simulink model "soc_WLAN_fpga"  (R2024b)
settings: Solver=FixedStepDiscrete  StartTime=0.0  StopTime=stopTime  RelTol=1e-3
PreLoadFcn:
  | addpath(fullfile(matlabroot,'toolbox','whdl','whdlexamples','whdlexamples'));
InitFcn:
  | addpath(fullfile(matlabroot,'toolbox','whdl','whdlexamples','whdlexamples'));
model workspace (MAT data in the model file):
  socvcb : containers.Map (value not decoded)
undefined symbols (not defined in the file): Add, bitRatePerOfdmSym, chanBW, coe, cpLen, dataUpsampleFactor, DelayValMaxNsdMinusLastPilotSc, DescramblerInitialSeed, designMultirateFIR, fftLen, filterLatency, filterUpsampleFactor, Fs, Hd, HT_MFMCS0, HT_MFMCS1, HT_MFMCS2, HT_MFMCS3, HT_MFMCS4, HT_MFMCS5, HT_MFMCS6, HT_MFMCS7, HTUnUsedScInd, inputSamplingRate, interp_coeff, maxPilotRefCounterVale, maxPilotsRef, maxPilotsRefNonHT, Ncol_HT, Ncol_NonHT, noDataSubCarriers, Non_HTMCS0, Non_HTMCS1, Non_HTMCS2, Non_HTMCS3, Non_HTMCS4, Non_HTMCS5, Non_HTMCS6, Non_HTMCS7, Nrow_HT, Nrow_NonHT, numDSC_HT, numDSC_HT_vhtSigB, numDSC_NonHT, numDscHT, numDscNonHT, numOfBitsPerOFDMSym, numOfDataBitsPerOFDMSym, numPilots, numScHT, numSCS_HT, numSCS_NonHT, pnSeq, QAM, rxDownsampleFactor, secondPIdx_HT, secondPIdx_NonHT, Shift, VHTMCS0, VHTMCS1 ... (+7)
libraries: hdlsllib x267, simulink x210, dspsigops x22, whdlutilities x10, whdlmod x9, dsphdlfiltering2 x5, dsphdlmathfun2 x4, whdledac x3, hwlogicconnlib x2, commhdlcrc x2, dsphdlsigops2 x2
(part 12 of 14)

== system soc_WLAN_fpga/WLAN/WLAN HDL/WLAN_Tx_Rx/WLAN_Rx/WLANHDLReceiver/FrameFormatDetectionAndSignalRecovery/SignalBitRecovery/Deinterleaver Block/Read Logic/Generate Read Address/Read Address of Deinterleaver/Generate Read Address ==
  note: Compute read address
  blockLen : Inport
  enable : Inport  Port=2
  reset : Inport  Port=3
  Add : Sum
  Add1 : Sum  OutDataTypeStr=fixdt(0,nextpow2(maxBlkSize),0)
  Constant : Constant  OutDataTypeStr=fixdt(0,1,0)  SampleTime=-1
  Constant1 : Constant  Value=nColumns-2  OutDataTypeStr=Inherit: Inherit via back propagation  SampleTime=-1
  Constant2 : Constant  Value=nColumns  OutDataTypeStr=fixdt(0,nextpow2(nColumns+1),0)  SampleTime=-1
  Constant4 : Constant  Value=nColumns  OutDataTypeStr=Inherit: Inherit via back propagation  SampleTime=-1
  Delay{,4..6,10..12,14..16} (10 alike) : Delay  DelayLength=1
  Delay{1..3,13} (4 alike) : Delay
  Divide : Product  Inputs=*/  OutDataTypeStr=fixdt(0,nextpow2(maxNRows+1),0)  RndMeth=Zero  SaturateOnIntegerOverflow=on
  From : From
  Goto : Goto
  HDL Counter2 : hdlsllib/Sources/HDL Counter  CountType=Count limited  CountInit=0  CountStep=1  CountMax=maxBlkSize  CountFromType=Initial value  CountFrom=0  CountResetPort=on  CountLoadPort=off  CountEnbPort=on  CountDirPort=off  CountHitOutputPort=off  CountDataType=Unsigned  CountWordLen=nextpow2(maxBlkSize+1)  CountFracLen=0  CountSampTime=1
  Logical Operator : Logic  Operator=OR  IconShape=distinctive  AllPortsSameDT=off  OutDataTypeStr=boolean
  Logical Operator1 : Logic  IconShape=distinctive  AllPortsSameDT=off  OutDataTypeStr=boolean
  Product : Product  OutDataTypeStr=fixdt(0,nextpow2(maxBlkSize),0)
  Relational Operator : RelationalOperator  Operator===  OutDataTypeStr=boolean  InputSameDT=off
  Relational Operator1 : RelationalOperator  OutDataTypeStr=boolean  InputSameDT=off
  Switch : Switch  Criteria=u2 ~= 0  SaturateOnIntegerOverflow=off  InputSameDT=off
  colCounter : hdlsllib/Sources/HDL Counter  CountType=Count limited  CountInit=0  CountStep=1  CountMax=maxNRows -1  CountFromType=Initial value  CountFrom=0  CountResetPort=on  CountLoadPort=off  CountEnbPort=on  CountDirPort=off  CountHitOutputPort=off  CountDataType=Unsigned  CountWordLen=nextpow2(maxNRows)  CountFracLen=0  CountSampTime=1
  rowCounter : hdlsllib/Sources/HDL Counter  CountType=Count limited  CountInit=0  CountStep=1  CountMax=nColumns -1  CountFromType=Initial value  CountFrom=0  CountResetPort=on  CountLoadPort=off  CountEnbPort=on  CountDirPort=off  CountHitOutputPort=off  CountDataType=Unsigned  CountWordLen=nextpow2(nColumns+1)  CountFracLen=0  CountSampTime=1
  blockDataCount : Outport
  currentAddr : Outport  Port=2
  wires:
  Relational Operator1/1 -> Logical Operator1/1
  HDL Counter2/1 -> Goto/1, Relational Operator1/2
  reset/1 -> Delay15/1, HDL Counter2/1
  Logical Operator/1 -> rowCounter/1
  Delay/1 -> Logical Operator/1, colCounter/2
  Relational Operator/1 -> Delay/1
  Constant/1 -> Add/2
  blockLen/1 -> Relational Operator1/1, Add/1
  enable/1 -> Logical Operator1/2, HDL Counter2/2
  rowCounter/1 -> Delay1/1, Relational Operator/2  "rowIndex"
  colCounter/1 -> Delay2/1  "colIndex"
  Add1/1 -> Delay6/1
  Product/1 -> Delay5/1
  Delay2/1 -> Delay4/1
  Delay4/1 -> Add1/2
  Delay5/1 -> Add1/1
  Delay15/1 -> colCounter/1, Logical Operator/2
  Delay16/1 -> Switch/2, rowCounter/2
  Delay13/1 -> Delay14/1
  Delay14/1 -> Delay11/1
  Delay12/1 -> Delay13/1
  Delay6/1 -> currentAddr/1
  Delay11/1 -> blockDataCount/1
  Add/1 -> Delay10/1
  From/1 -> Delay12/1
  Logical Operator1/1 -> Delay16/1
  Divide/1 -> Delay3/1
  Delay10/1 -> Divide/1
  Constant2/1 -> Divide/2
  Switch/1 -> Relational Operator/1
  Constant1/1 -> Switch/1
  Constant4/1 -> Switch/3
  Delay1/1 -> Product/2
  Delay3/1 -> Product/1

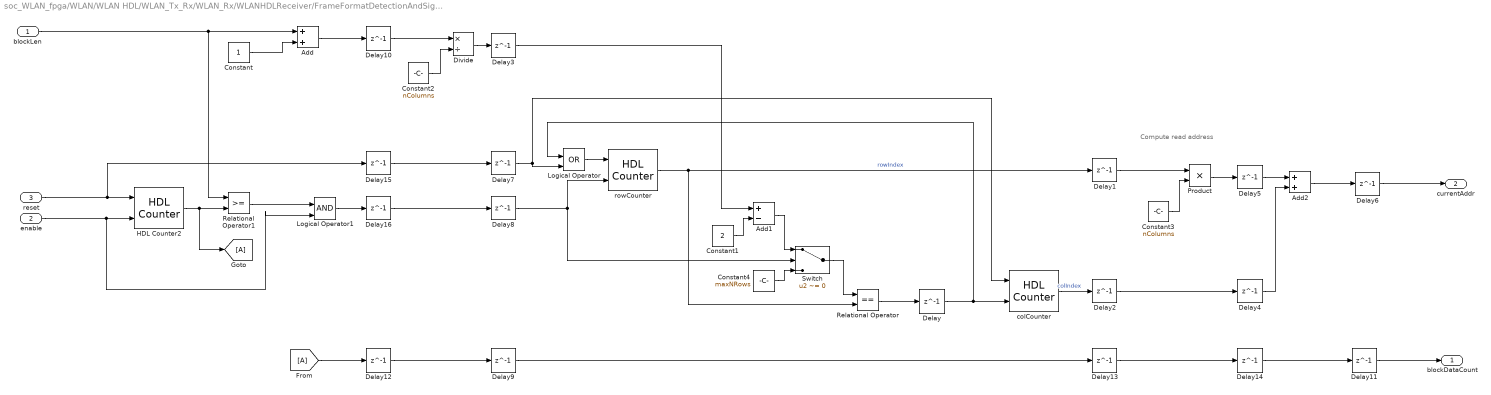
== system soc_WLAN_fpga/WLAN/WLAN HDL/WLAN_Tx_Rx/WLAN_Rx/WLANHDLReceiver/FrameFormatDetectionAndSignalRecovery/SignalBitRecovery/Deinterleaver Block/Read Logic/Generate Read Address/Read Address of Interleaver/Generate Read Address ==
  note: Compute read address
  blockLen : Inport
  enable : Inport  Port=2
  reset : Inport  Port=3
  Add : Sum
  Add1 : Sum  Inputs=+-  OutDataTypeStr=Inherit: Inherit via back propagation
  Add2 : Sum  OutDataTypeStr=fixdt(0,nextpow2(maxBlkSize),0)
  Constant : Constant  OutDataTypeStr=fixdt(0,1,0)  SampleTime=-1
  Constant1 : Constant  Value=2  OutDataTypeStr=fixdt(0,2,0)  SampleTime=-1
  Constant2 : Constant  Value=nColumns  OutDataTypeStr=fixdt(0,nextpow2(nColumns+1),0)  SampleTime=-1
  Constant3 : Constant  Value=nColumns  OutDataTypeStr=fixdt(0,nextpow2(nColumns+1),0)  SampleTime=-1
  Constant4 : Constant  Value=maxNRows  OutDataTypeStr=Inherit: Inherit via back propagation  SampleTime=-1
  Delay{,1..16} (17 alike) : Delay  DelayLength=1
  Divide : Product  Inputs=*/  OutDataTypeStr=fixdt(0,nextpow2(maxNRows+1),0)  RndMeth=Zero  SaturateOnIntegerOverflow=on
  From : From
  Goto : Goto
  HDL Counter2 : hdlsllib/Sources/HDL Counter  CountType=Count limited  CountInit=0  CountStep=1  CountMax=maxBlkSize  CountFromType=Initial value  CountFrom=0  CountResetPort=on  CountLoadPort=off  CountEnbPort=on  CountDirPort=off  CountHitOutputPort=off  CountDataType=Unsigned  CountWordLen=nextpow2(maxBlkSize+1)  CountFracLen=0  CountSampTime=1
  Logical Operator : Logic  Operator=OR  IconShape=distinctive  AllPortsSameDT=off  OutDataTypeStr=boolean
  Logical Operator1 : Logic  IconShape=distinctive  AllPortsSameDT=off  OutDataTypeStr=boolean
  Product : Product  OutDataTypeStr=fixdt(0,nextpow2(maxBlkSize),0)
  Relational Operator : RelationalOperator  Operator===  OutDataTypeStr=boolean  InputSameDT=off
  Relational Operator1 : RelationalOperator  OutDataTypeStr=boolean  InputSameDT=off
  Switch : Switch  Criteria=u2 ~= 0  SaturateOnIntegerOverflow=off  InputSameDT=off
  colCounter : hdlsllib/Sources/HDL Counter  CountType=Count limited  CountInit=0  CountStep=1  CountMax=nColumns -1  CountFromType=Initial value  CountFrom=0  CountResetPort=on  CountLoadPort=off  CountEnbPort=on  CountDirPort=off  CountHitOutputPort=off  CountDataType=Unsigned  CountWordLen=nextpow2(nColumns)  CountFracLen=0  CountSampTime=1
  rowCounter : hdlsllib/Sources/HDL Counter  CountType=Count limited  CountInit=0  CountStep=1  CountMax=maxNRows -1  CountFromType=Initial value  CountFrom=0  CountResetPort=on  CountLoadPort=off  CountEnbPort=on  CountDirPort=off  CountHitOutputPort=off  CountDataType=Unsigned  CountWordLen=nextpow2(maxNRows+1)  CountFracLen=0  CountSampTime=1
  blockDataCount : Outport
  currentAddr : Outport  Port=2
  wires:
  Constant3/1 -> Product/2
  Delay9/1 -> Delay13/1
  Delay8/1 -> rowCounter/2, Switch/2
  Delay7/1 -> Logical Operator/2, colCounter/1
  Delay3/1 -> Add1/1
  Delay1/1 -> Product/1
  Add1/1 -> Switch/1
  Constant1/1 -> Add1/2
  Divide/1 -> Delay3/1
  Constant4/1 -> Switch/3
  Switch/1 -> Relational Operator/1
  Constant2/1 -> Divide/2
  Delay10/1 -> Divide/1
  Logical Operator1/1 -> Delay16/1
  From/1 -> Delay12/1
  Add/1 -> Delay10/1
  Delay11/1 -> blockDataCount/1
  Delay6/1 -> currentAddr/1
  Delay12/1 -> Delay9/1
  Delay14/1 -> Delay11/1
  Delay13/1 -> Delay14/1
  Delay16/1 -> Delay8/1
  Delay15/1 -> Delay7/1
  Delay5/1 -> Add2/1
  Delay4/1 -> Add2/2
  Delay2/1 -> Delay4/1
  Product/1 -> Delay5/1
  Add2/1 -> Delay6/1
  colCounter/1 -> Delay2/1  "colIndex"
  rowCounter/1 -> Delay1/1, Relational Operator/2  "rowIndex"
  enable/1 -> HDL Counter2/2, Logical Operator1/2
  blockLen/1 -> Add/1, Relational Operator1/1
  Constant/1 -> Add/2
  Relational Operator/1 -> Delay/1
  Delay/1 -> colCounter/2, Logical Operator/1
  Logical Operator/1 -> rowCounter/1
  reset/1 -> HDL Counter2/1, Delay15/1
  HDL Counter2/1 -> Relational Operator1/2, Goto/1
  Relational Operator1/1 -> Logical Operator1/1

== system soc_WLAN_fpga/WLAN/WLAN HDL/WLAN_Tx_Rx/WLAN_Rx/WLANHDLReceiver/DataRecovery/Deinterleaver/DeInterleaver_HT/Stage 2 16QAM /Read Logic/Generate Read Address/Read Address of Deinterleaver/Generate Read Address ==
  note: Compute read address
  blockLen : Inport
  enable : Inport  Port=2
  reset : Inport  Port=3
  Add : Sum
  Add1 : Sum  OutDataTypeStr=fixdt(0,nextpow2(maxBlkSize),0)
  Constant : Constant  OutDataTypeStr=fixdt(0,1,0)  SampleTime=-1
  Constant1 : Constant  Value=nColumns-2  OutDataTypeStr=Inherit: Inherit via back propagation  SampleTime=-1
  Constant2 : Constant  Value=nColumns  OutDataTypeStr=fixdt(0,nextpow2(nColumns+1),0)  SampleTime=-1
  Constant4 : Constant  Value=nColumns  OutDataTypeStr=Inherit: Inherit via back propagation  SampleTime=-1
  Delay{,4..6,10..12,14..16} (10 alike) : Delay  DelayLength=1
  Delay{1..3,13} (4 alike) : Delay
  Divide : Product  Inputs=*/  OutDataTypeStr=fixdt(0,nextpow2(maxNRows+1),0)  RndMeth=Zero  SaturateOnIntegerOverflow=on
  From : From
  Goto : Goto
  HDL Counter2 : hdlsllib/Sources/HDL Counter  CountType=Count limited  CountInit=0  CountStep=1  CountMax=maxBlkSize  CountFromType=Initial value  CountFrom=0  CountResetPort=on  CountLoadPort=off  CountEnbPort=on  CountDirPort=off  CountHitOutputPort=off  CountDataType=Unsigned  CountWordLen=nextpow2(maxBlkSize+1)  CountFracLen=0  CountSampTime=1
  Logical Operator : Logic  Operator=OR  IconShape=distinctive  AllPortsSameDT=off  OutDataTypeStr=boolean
  Logical Operator1 : Logic  IconShape=distinctive  AllPortsSameDT=off  OutDataTypeStr=boolean
  Product : Product  OutDataTypeStr=fixdt(0,nextpow2(maxBlkSize),0)
  Relational Operator : RelationalOperator  Operator===  OutDataTypeStr=boolean  InputSameDT=off
  Relational Operator1 : RelationalOperator  OutDataTypeStr=boolean  InputSameDT=off
  Switch : Switch  Criteria=u2 ~= 0  SaturateOnIntegerOverflow=off  InputSameDT=off
  colCounter : hdlsllib/Sources/HDL Counter  CountType=Count limited  CountInit=0  CountStep=1  CountMax=maxNRows -1  CountFromType=Initial value  CountFrom=0  CountResetPort=on  CountLoadPort=off  CountEnbPort=on  CountDirPort=off  CountHitOutputPort=off  CountDataType=Unsigned  CountWordLen=nextpow2(maxNRows)  CountFracLen=0  CountSampTime=1
  rowCounter : hdlsllib/Sources/HDL Counter  CountType=Count limited  CountInit=0  CountStep=1  CountMax=nColumns -1  CountFromType=Initial value  CountFrom=0  CountResetPort=on  CountLoadPort=off  CountEnbPort=on  CountDirPort=off  CountHitOutputPort=off  CountDataType=Unsigned  CountWordLen=nextpow2(nColumns+1)  CountFracLen=0  CountSampTime=1
  blockDataCount : Outport
  currentAddr : Outport  Port=2
  wires:
  Relational Operator1/1 -> Logical Operator1/1
  HDL Counter2/1 -> Goto/1, Relational Operator1/2
  reset/1 -> Delay15/1, HDL Counter2/1
  Logical Operator/1 -> rowCounter/1
  Delay/1 -> Logical Operator/1, colCounter/2
  Relational Operator/1 -> Delay/1
  Constant/1 -> Add/2
  blockLen/1 -> Relational Operator1/1, Add/1
  enable/1 -> Logical Operator1/2, HDL Counter2/2
  rowCounter/1 -> Delay1/1, Relational Operator/2  "rowIndex"
  colCounter/1 -> Delay2/1  "colIndex"
  Add1/1 -> Delay6/1
  Product/1 -> Delay5/1
  Delay2/1 -> Delay4/1
  Delay4/1 -> Add1/2
  Delay5/1 -> Add1/1
  Delay15/1 -> colCounter/1, Logical Operator/2
  Delay16/1 -> Switch/2, rowCounter/2
  Delay13/1 -> Delay14/1
  Delay14/1 -> Delay11/1
  Delay12/1 -> Delay13/1
  Delay6/1 -> currentAddr/1
  Delay11/1 -> blockDataCount/1
  Add/1 -> Delay10/1
  From/1 -> Delay12/1
  Logical Operator1/1 -> Delay16/1
  Divide/1 -> Delay3/1
  Delay10/1 -> Divide/1
  Constant2/1 -> Divide/2
  Switch/1 -> Relational Operator/1
  Constant1/1 -> Switch/1
  Constant4/1 -> Switch/3
  Delay1/1 -> Product/2
  Delay3/1 -> Product/1

== system soc_WLAN_fpga/WLAN/WLAN HDL/WLAN_Tx_Rx/WLAN_Rx/WLANHDLReceiver/DataRecovery/Deinterleaver/DeInterleaver_HT/Stage 2 16QAM /Read Logic/Generate Read Address/Read Address of Interleaver/Generate Read Address ==
  note: Compute read address
  blockLen : Inport
  enable : Inport  Port=2
  reset : Inport  Port=3
  Add : Sum
  Add1 : Sum  Inputs=+-  OutDataTypeStr=Inherit: Inherit via back propagation
  Add2 : Sum  OutDataTypeStr=fixdt(0,nextpow2(maxBlkSize),0)
  Constant : Constant  OutDataTypeStr=fixdt(0,1,0)  SampleTime=-1
  Constant1 : Constant  Value=2  OutDataTypeStr=fixdt(0,2,0)  SampleTime=-1
  Constant2 : Constant  Value=nColumns  OutDataTypeStr=fixdt(0,nextpow2(nColumns+1),0)  SampleTime=-1
  Constant3 : Constant  Value=nColumns  OutDataTypeStr=fixdt(0,nextpow2(nColumns+1),0)  SampleTime=-1
  Constant4 : Constant  Value=maxNRows  OutDataTypeStr=Inherit: Inherit via back propagation  SampleTime=-1
  Delay{,1..16} (17 alike) : Delay  DelayLength=1
  Divide : Product  Inputs=*/  OutDataTypeStr=fixdt(0,nextpow2(maxNRows+1),0)  RndMeth=Zero  SaturateOnIntegerOverflow=on
  From : From
  Goto : Goto
  HDL Counter2 : hdlsllib/Sources/HDL Counter  CountType=Count limited  CountInit=0  CountStep=1  CountMax=maxBlkSize  CountFromType=Initial value  CountFrom=0  CountResetPort=on  CountLoadPort=off  CountEnbPort=on  CountDirPort=off  CountHitOutputPort=off  CountDataType=Unsigned  CountWordLen=nextpow2(maxBlkSize+1)  CountFracLen=0  CountSampTime=1
  Logical Operator : Logic  Operator=OR  IconShape=distinctive  AllPortsSameDT=off  OutDataTypeStr=boolean
  Logical Operator1 : Logic  IconShape=distinctive  AllPortsSameDT=off  OutDataTypeStr=boolean
  Product : Product  OutDataTypeStr=fixdt(0,nextpow2(maxBlkSize),0)
  Relational Operator : RelationalOperator  Operator===  OutDataTypeStr=boolean  InputSameDT=off
  Relational Operator1 : RelationalOperator  OutDataTypeStr=boolean  InputSameDT=off
  Switch : Switch  Criteria=u2 ~= 0  SaturateOnIntegerOverflow=off  InputSameDT=off
  colCounter : hdlsllib/Sources/HDL Counter  CountType=Count limited  CountInit=0  CountStep=1  CountMax=nColumns -1  CountFromType=Initial value  CountFrom=0  CountResetPort=on  CountLoadPort=off  CountEnbPort=on  CountDirPort=off  CountHitOutputPort=off  CountDataType=Unsigned  CountWordLen=nextpow2(nColumns)  CountFracLen=0  CountSampTime=1
  rowCounter : hdlsllib/Sources/HDL Counter  CountType=Count limited  CountInit=0  CountStep=1  CountMax=maxNRows -1  CountFromType=Initial value  CountFrom=0  CountResetPort=on  CountLoadPort=off  CountEnbPort=on  CountDirPort=off  CountHitOutputPort=off  CountDataType=Unsigned  CountWordLen=nextpow2(maxNRows+1)  CountFracLen=0  CountSampTime=1
  blockDataCount : Outport
  currentAddr : Outport  Port=2
  wires:
  Constant3/1 -> Product/2
  Delay9/1 -> Delay13/1
  Delay8/1 -> rowCounter/2, Switch/2
  Delay7/1 -> Logical Operator/2, colCounter/1
  Delay3/1 -> Add1/1
  Delay1/1 -> Product/1
  Add1/1 -> Switch/1
  Constant1/1 -> Add1/2
  Divide/1 -> Delay3/1
  Constant4/1 -> Switch/3
  Switch/1 -> Relational Operator/1
  Constant2/1 -> Divide/2
  Delay10/1 -> Divide/1
  Logical Operator1/1 -> Delay16/1
  From/1 -> Delay12/1
  Add/1 -> Delay10/1
  Delay11/1 -> blockDataCount/1
  Delay6/1 -> currentAddr/1
  Delay12/1 -> Delay9/1
  Delay14/1 -> Delay11/1
  Delay13/1 -> Delay14/1
  Delay16/1 -> Delay8/1
  Delay15/1 -> Delay7/1
  Delay5/1 -> Add2/1
  Delay4/1 -> Add2/2
  Delay2/1 -> Delay4/1
  Product/1 -> Delay5/1
  Add2/1 -> Delay6/1
  colCounter/1 -> Delay2/1  "colIndex"
  rowCounter/1 -> Delay1/1, Relational Operator/2  "rowIndex"
  enable/1 -> HDL Counter2/2, Logical Operator1/2
  blockLen/1 -> Add/1, Relational Operator1/1
  Constant/1 -> Add/2
  Relational Operator/1 -> Delay/1
  Delay/1 -> colCounter/2, Logical Operator/1
  Logical Operator/1 -> rowCounter/1
  reset/1 -> HDL Counter2/1, Delay15/1
  HDL Counter2/1 -> Relational Operator1/2, Goto/1
  Relational Operator1/1 -> Logical Operator1/1

== system soc_WLAN_fpga/WLAN/WLAN HDL/WLAN_Tx_Rx/WLAN_Rx/WLANHDLReceiver/DataRecovery/Deinterleaver/DeInterleaver_HT/Stage 2 64QAM/Read Logic/Generate Read Address/Read Address of Deinterleaver/Generate Read Address ==
  note: Compute read address
  blockLen : Inport
  enable : Inport  Port=2
  reset : Inport  Port=3
  Add : Sum
  Add1 : Sum  OutDataTypeStr=fixdt(0,nextpow2(maxBlkSize),0)
  Constant : Constant  OutDataTypeStr=fixdt(0,1,0)  SampleTime=-1
  Constant1 : Constant  Value=nColumns-2  OutDataTypeStr=Inherit: Inherit via back propagation  SampleTime=-1
  Constant2 : Constant  Value=nColumns  OutDataTypeStr=fixdt(0,nextpow2(nColumns+1),0)  SampleTime=-1
  Constant4 : Constant  Value=nColumns  OutDataTypeStr=Inherit: Inherit via back propagation  SampleTime=-1
  Delay{,4..6,10..12,14..16} (10 alike) : Delay  DelayLength=1
  Delay{1..3,13} (4 alike) : Delay
  Divide : Product  Inputs=*/  OutDataTypeStr=fixdt(0,nextpow2(maxNRows+1),0)  RndMeth=Zero  SaturateOnIntegerOverflow=on
  From : From
  Goto : Goto
  HDL Counter2 : hdlsllib/Sources/HDL Counter  CountType=Count limited  CountInit=0  CountStep=1  CountMax=maxBlkSize  CountFromType=Initial value  CountFrom=0  CountResetPort=on  CountLoadPort=off  CountEnbPort=on  CountDirPort=off  CountHitOutputPort=off  CountDataType=Unsigned  CountWordLen=nextpow2(maxBlkSize+1)  CountFracLen=0  CountSampTime=1
  Logical Operator : Logic  Operator=OR  IconShape=distinctive  AllPortsSameDT=off  OutDataTypeStr=boolean
  Logical Operator1 : Logic  IconShape=distinctive  AllPortsSameDT=off  OutDataTypeStr=boolean
  Product : Product  OutDataTypeStr=fixdt(0,nextpow2(maxBlkSize),0)
  Relational Operator : RelationalOperator  Operator===  OutDataTypeStr=boolean  InputSameDT=off
  Relational Operator1 : RelationalOperator  OutDataTypeStr=boolean  InputSameDT=off
  Switch : Switch  Criteria=u2 ~= 0  SaturateOnIntegerOverflow=off  InputSameDT=off
  colCounter : hdlsllib/Sources/HDL Counter  CountType=Count limited  CountInit=0  CountStep=1  CountMax=maxNRows -1  CountFromType=Initial value  CountFrom=0  CountResetPort=on  CountLoadPort=off  CountEnbPort=on  CountDirPort=off  CountHitOutputPort=off  CountDataType=Unsigned  CountWordLen=nextpow2(maxNRows)  CountFracLen=0  CountSampTime=1
  rowCounter : hdlsllib/Sources/HDL Counter  CountType=Count limited  CountInit=0  CountStep=1  CountMax=nColumns -1  CountFromType=Initial value  CountFrom=0  CountResetPort=on  CountLoadPort=off  CountEnbPort=on  CountDirPort=off  CountHitOutputPort=off  CountDataType=Unsigned  CountWordLen=nextpow2(nColumns+1)  CountFracLen=0  CountSampTime=1
  blockDataCount : Outport
  currentAddr : Outport  Port=2
  wires:
  Relational Operator1/1 -> Logical Operator1/1
  HDL Counter2/1 -> Goto/1, Relational Operator1/2
  reset/1 -> Delay15/1, HDL Counter2/1
  Logical Operator/1 -> rowCounter/1
  Delay/1 -> Logical Operator/1, colCounter/2
  Relational Operator/1 -> Delay/1
  Constant/1 -> Add/2
  blockLen/1 -> Relational Operator1/1, Add/1
  enable/1 -> Logical Operator1/2, HDL Counter2/2
  rowCounter/1 -> Delay1/1, Relational Operator/2  "rowIndex"
  colCounter/1 -> Delay2/1  "colIndex"
  Add1/1 -> Delay6/1
  Product/1 -> Delay5/1
  Delay2/1 -> Delay4/1
  Delay4/1 -> Add1/2
  Delay5/1 -> Add1/1
  Delay15/1 -> colCounter/1, Logical Operator/2
  Delay16/1 -> Switch/2, rowCounter/2
  Delay13/1 -> Delay14/1
  Delay14/1 -> Delay11/1
  Delay12/1 -> Delay13/1
  Delay6/1 -> currentAddr/1
  Delay11/1 -> blockDataCount/1
  Add/1 -> Delay10/1
  From/1 -> Delay12/1
  Logical Operator1/1 -> Delay16/1
  Divide/1 -> Delay3/1
  Delay10/1 -> Divide/1
  Constant2/1 -> Divide/2
  Switch/1 -> Relational Operator/1
  Constant1/1 -> Switch/1
  Constant4/1 -> Switch/3
  Delay1/1 -> Product/2
  Delay3/1 -> Product/1

== system soc_WLAN_fpga/WLAN/WLAN HDL/WLAN_Tx_Rx/WLAN_Rx/WLANHDLReceiver/DataRecovery/Deinterleaver/DeInterleaver_HT/Stage 2 64QAM/Read Logic/Generate Read Address/Read Address of Interleaver/Generate Read Address ==
  note: Compute read address
  blockLen : Inport
  enable : Inport  Port=2
  reset : Inport  Port=3
  Add : Sum
  Add1 : Sum  Inputs=+-  OutDataTypeStr=Inherit: Inherit via back propagation
  Add2 : Sum  OutDataTypeStr=fixdt(0,nextpow2(maxBlkSize),0)
  Constant : Constant  OutDataTypeStr=fixdt(0,1,0)  SampleTime=-1
  Constant1 : Constant  Value=2  OutDataTypeStr=fixdt(0,2,0)  SampleTime=-1
  Constant2 : Constant  Value=nColumns  OutDataTypeStr=fixdt(0,nextpow2(nColumns+1),0)  SampleTime=-1
  Constant3 : Constant  Value=nColumns  OutDataTypeStr=fixdt(0,nextpow2(nColumns+1),0)  SampleTime=-1
  Constant4 : Constant  Value=maxNRows  OutDataTypeStr=Inherit: Inherit via back propagation  SampleTime=-1
  Delay{,1..16} (17 alike) : Delay  DelayLength=1
  Divide : Product  Inputs=*/  OutDataTypeStr=fixdt(0,nextpow2(maxNRows+1),0)  RndMeth=Zero  SaturateOnIntegerOverflow=on
  From : From
  Goto : Goto
  HDL Counter2 : hdlsllib/Sources/HDL Counter  CountType=Count limited  CountInit=0  CountStep=1  CountMax=maxBlkSize  CountFromType=Initial value  CountFrom=0  CountResetPort=on  CountLoadPort=off  CountEnbPort=on  CountDirPort=off  CountHitOutputPort=off  CountDataType=Unsigned  CountWordLen=nextpow2(maxBlkSize+1)  CountFracLen=0  CountSampTime=1
  Logical Operator : Logic  Operator=OR  IconShape=distinctive  AllPortsSameDT=off  OutDataTypeStr=boolean
  Logical Operator1 : Logic  IconShape=distinctive  AllPortsSameDT=off  OutDataTypeStr=boolean
  Product : Product  OutDataTypeStr=fixdt(0,nextpow2(maxBlkSize),0)
  Relational Operator : RelationalOperator  Operator===  OutDataTypeStr=boolean  InputSameDT=off
  Relational Operator1 : RelationalOperator  OutDataTypeStr=boolean  InputSameDT=off
  Switch : Switch  Criteria=u2 ~= 0  SaturateOnIntegerOverflow=off  InputSameDT=off
  colCounter : hdlsllib/Sources/HDL Counter  CountType=Count limited  CountInit=0  CountStep=1  CountMax=nColumns -1  CountFromType=Initial value  CountFrom=0  CountResetPort=on  CountLoadPort=off  CountEnbPort=on  CountDirPort=off  CountHitOutputPort=off  CountDataType=Unsigned  CountWordLen=nextpow2(nColumns)  CountFracLen=0  CountSampTime=1
  rowCounter : hdlsllib/Sources/HDL Counter  CountType=Count limited  CountInit=0  CountStep=1  CountMax=maxNRows -1  CountFromType=Initial value  CountFrom=0  CountResetPort=on  CountLoadPort=off  CountEnbPort=on  CountDirPort=off  CountHitOutputPort=off  CountDataType=Unsigned  CountWordLen=nextpow2(maxNRows+1)  CountFracLen=0  CountSampTime=1
  blockDataCount : Outport
  currentAddr : Outport  Port=2
  wires:
  Constant3/1 -> Product/2
  Delay9/1 -> Delay13/1
  Delay8/1 -> rowCounter/2, Switch/2
  Delay7/1 -> Logical Operator/2, colCounter/1
  Delay3/1 -> Add1/1
  Delay1/1 -> Product/1
  Add1/1 -> Switch/1
  Constant1/1 -> Add1/2
  Divide/1 -> Delay3/1
  Constant4/1 -> Switch/3
  Switch/1 -> Relational Operator/1
  Constant2/1 -> Divide/2
  Delay10/1 -> Divide/1
  Logical Operator1/1 -> Delay16/1
  From/1 -> Delay12/1
  Add/1 -> Delay10/1
  Delay11/1 -> blockDataCount/1
  Delay6/1 -> currentAddr/1
  Delay12/1 -> Delay9/1
  Delay14/1 -> Delay11/1
  Delay13/1 -> Delay14/1
  Delay16/1 -> Delay8/1
  Delay15/1 -> Delay7/1
  Delay5/1 -> Add2/1
  Delay4/1 -> Add2/2
  Delay2/1 -> Delay4/1
  Product/1 -> Delay5/1
  Add2/1 -> Delay6/1
  colCounter/1 -> Delay2/1  "colIndex"
  rowCounter/1 -> Delay1/1, Relational Operator/2  "rowIndex"
  enable/1 -> HDL Counter2/2, Logical Operator1/2
  blockLen/1 -> Add/1, Relational Operator1/1
  Constant/1 -> Add/2
  Relational Operator/1 -> Delay/1
  Delay/1 -> colCounter/2, Logical Operator/1
  Logical Operator/1 -> rowCounter/1
  reset/1 -> HDL Counter2/1, Delay15/1
  HDL Counter2/1 -> Relational Operator1/2, Goto/1
  Relational Operator1/1 -> Logical Operator1/1

== system soc_WLAN_fpga/WLAN/WLAN HDL/WLAN_Tx_Rx/WLAN_Rx/WLANHDLReceiver/DataRecovery/Deinterleaver/DeInterleaver_HT/Stage 2 BPSK/Read Logic/Generate Read Address/Read Address of Deinterleaver/Generate Read Address ==
  note: Compute read address
  blockLen : Inport
  enable : Inport  Port=2
  reset : Inport  Port=3
  Add : Sum
  Add1 : Sum  OutDataTypeStr=fixdt(0,nextpow2(maxBlkSize),0)
  Constant : Constant  OutDataTypeStr=fixdt(0,1,0)  SampleTime=-1
  Constant1 : Constant  Value=nColumns-2  OutDataTypeStr=Inherit: Inherit via back propagation  SampleTime=-1
  Constant2 : Constant  Value=nColumns  OutDataTypeStr=fixdt(0,nextpow2(nColumns+1),0)  SampleTime=-1
  Constant4 : Constant  Value=nColumns  OutDataTypeStr=Inherit: Inherit via back propagation  SampleTime=-1
  Delay{,4..6,10..12,14..16} (10 alike) : Delay  DelayLength=1
  Delay{1..3,13} (4 alike) : Delay
  Divide : Product  Inputs=*/  OutDataTypeStr=fixdt(0,nextpow2(maxNRows+1),0)  RndMeth=Zero  SaturateOnIntegerOverflow=on
  From : From
  Goto : Goto
  HDL Counter2 : hdlsllib/Sources/HDL Counter  CountType=Count limited  CountInit=0  CountStep=1  CountMax=maxBlkSize  CountFromType=Initial value  CountFrom=0  CountResetPort=on  CountLoadPort=off  CountEnbPort=on  CountDirPort=off  CountHitOutputPort=off  CountDataType=Unsigned  CountWordLen=nextpow2(maxBlkSize+1)  CountFracLen=0  CountSampTime=1
  Logical Operator : Logic  Operator=OR  IconShape=distinctive  AllPortsSameDT=off  OutDataTypeStr=boolean
  Logical Operator1 : Logic  IconShape=distinctive  AllPortsSameDT=off  OutDataTypeStr=boolean
  Product : Product  OutDataTypeStr=fixdt(0,nextpow2(maxBlkSize),0)
  Relational Operator : RelationalOperator  Operator===  OutDataTypeStr=boolean  InputSameDT=off
  Relational Operator1 : RelationalOperator  OutDataTypeStr=boolean  InputSameDT=off
  Switch : Switch  Criteria=u2 ~= 0  SaturateOnIntegerOverflow=off  InputSameDT=off
  colCounter : hdlsllib/Sources/HDL Counter  CountType=Count limited  CountInit=0  CountStep=1  CountMax=maxNRows -1  CountFromType=Initial value  CountFrom=0  CountResetPort=on  CountLoadPort=off  CountEnbPort=on  CountDirPort=off  CountHitOutputPort=off  CountDataType=Unsigned  CountWordLen=nextpow2(maxNRows)  CountFracLen=0  CountSampTime=1
  rowCounter : hdlsllib/Sources/HDL Counter  CountType=Count limited  CountInit=0  CountStep=1  CountMax=nColumns -1  CountFromType=Initial value  CountFrom=0  CountResetPort=on  CountLoadPort=off  CountEnbPort=on  CountDirPort=off  CountHitOutputPort=off  CountDataType=Unsigned  CountWordLen=nextpow2(nColumns+1)  CountFracLen=0  CountSampTime=1
  blockDataCount : Outport
  currentAddr : Outport  Port=2
  wires:
  Relational Operator1/1 -> Logical Operator1/1
  HDL Counter2/1 -> Goto/1, Relational Operator1/2
  reset/1 -> Delay15/1, HDL Counter2/1
  Logical Operator/1 -> rowCounter/1
  Delay/1 -> Logical Operator/1, colCounter/2
  Relational Operator/1 -> Delay/1
  Constant/1 -> Add/2
  blockLen/1 -> Relational Operator1/1, Add/1
  enable/1 -> Logical Operator1/2, HDL Counter2/2
  rowCounter/1 -> Delay1/1, Relational Operator/2  "rowIndex"
  colCounter/1 -> Delay2/1  "colIndex"
  Add1/1 -> Delay6/1
  Product/1 -> Delay5/1
  Delay2/1 -> Delay4/1
  Delay4/1 -> Add1/2
  Delay5/1 -> Add1/1
  Delay15/1 -> colCounter/1, Logical Operator/2
  Delay16/1 -> Switch/2, rowCounter/2
  Delay13/1 -> Delay14/1
  Delay14/1 -> Delay11/1
  Delay12/1 -> Delay13/1
  Delay6/1 -> currentAddr/1
  Delay11/1 -> blockDataCount/1
  Add/1 -> Delay10/1
  From/1 -> Delay12/1
  Logical Operator1/1 -> Delay16/1
  Divide/1 -> Delay3/1
  Delay10/1 -> Divide/1
  Constant2/1 -> Divide/2
  Switch/1 -> Relational Operator/1
  Constant1/1 -> Switch/1
  Constant4/1 -> Switch/3
  Delay1/1 -> Product/2
  Delay3/1 -> Product/1

== system soc_WLAN_fpga/WLAN/WLAN HDL/WLAN_Tx_Rx/WLAN_Rx/WLANHDLReceiver/DataRecovery/Deinterleaver/DeInterleaver_HT/Stage 2 BPSK/Read Logic/Generate Read Address/Read Address of Interleaver/Generate Read Address ==
  note: Compute read address
  blockLen : Inport
  enable : Inport  Port=2
  reset : Inport  Port=3
  Add : Sum
  Add1 : Sum  Inputs=+-  OutDataTypeStr=Inherit: Inherit via back propagation
  Add2 : Sum  OutDataTypeStr=fixdt(0,nextpow2(maxBlkSize),0)
  Constant : Constant  OutDataTypeStr=fixdt(0,1,0)  SampleTime=-1
  Constant1 : Constant  Value=2  OutDataTypeStr=fixdt(0,2,0)  SampleTime=-1
  Constant2 : Constant  Value=nColumns  OutDataTypeStr=fixdt(0,nextpow2(nColumns+1),0)  SampleTime=-1
  Constant3 : Constant  Value=nColumns  OutDataTypeStr=fixdt(0,nextpow2(nColumns+1),0)  SampleTime=-1
  Constant4 : Constant  Value=maxNRows  OutDataTypeStr=Inherit: Inherit via back propagation  SampleTime=-1
  Delay{,1..16} (17 alike) : Delay  DelayLength=1
  Divide : Product  Inputs=*/  OutDataTypeStr=fixdt(0,nextpow2(maxNRows+1),0)  RndMeth=Zero  SaturateOnIntegerOverflow=on
  From : From
  Goto : Goto
  HDL Counter2 : hdlsllib/Sources/HDL Counter  CountType=Count limited  CountInit=0  CountStep=1  CountMax=maxBlkSize  CountFromType=Initial value  CountFrom=0  CountResetPort=on  CountLoadPort=off  CountEnbPort=on  CountDirPort=off  CountHitOutputPort=off  CountDataType=Unsigned  CountWordLen=nextpow2(maxBlkSize+1)  CountFracLen=0  CountSampTime=1
  Logical Operator : Logic  Operator=OR  IconShape=distinctive  AllPortsSameDT=off  OutDataTypeStr=boolean
  Logical Operator1 : Logic  IconShape=distinctive  AllPortsSameDT=off  OutDataTypeStr=boolean
  Product : Product  OutDataTypeStr=fixdt(0,nextpow2(maxBlkSize),0)
  Relational Operator : RelationalOperator  Operator===  OutDataTypeStr=boolean  InputSameDT=off
  Relational Operator1 : RelationalOperator  OutDataTypeStr=boolean  InputSameDT=off
  Switch : Switch  Criteria=u2 ~= 0  SaturateOnIntegerOverflow=off  InputSameDT=off
  colCounter : hdlsllib/Sources/HDL Counter  CountType=Count limited  CountInit=0  CountStep=1  CountMax=nColumns -1  CountFromType=Initial value  CountFrom=0  CountResetPort=on  CountLoadPort=off  CountEnbPort=on  CountDirPort=off  CountHitOutputPort=off  CountDataType=Unsigned  CountWordLen=nextpow2(nColumns)  CountFracLen=0  CountSampTime=1
  rowCounter : hdlsllib/Sources/HDL Counter  CountType=Count limited  CountInit=0  CountStep=1  CountMax=maxNRows -1  CountFromType=Initial value  CountFrom=0  CountResetPort=on  CountLoadPort=off  CountEnbPort=on  CountDirPort=off  CountHitOutputPort=off  CountDataType=Unsigned  CountWordLen=nextpow2(maxNRows+1)  CountFracLen=0  CountSampTime=1
  blockDataCount : Outport
  currentAddr : Outport  Port=2
  wires:
  Constant3/1 -> Product/2
  Delay9/1 -> Delay13/1
  Delay8/1 -> rowCounter/2, Switch/2
  Delay7/1 -> Logical Operator/2, colCounter/1
  Delay3/1 -> Add1/1
  Delay1/1 -> Product/1
  Add1/1 -> Switch/1
  Constant1/1 -> Add1/2
  Divide/1 -> Delay3/1
  Constant4/1 -> Switch/3
  Switch/1 -> Relational Operator/1
  Constant2/1 -> Divide/2
  Delay10/1 -> Divide/1
  Logical Operator1/1 -> Delay16/1
  From/1 -> Delay12/1
  Add/1 -> Delay10/1
  Delay11/1 -> blockDataCount/1
  Delay6/1 -> currentAddr/1
  Delay12/1 -> Delay9/1
  Delay14/1 -> Delay11/1
  Delay13/1 -> Delay14/1
  Delay16/1 -> Delay8/1
  Delay15/1 -> Delay7/1
  Delay5/1 -> Add2/1
  Delay4/1 -> Add2/2
  Delay2/1 -> Delay4/1
  Product/1 -> Delay5/1
  Add2/1 -> Delay6/1
  colCounter/1 -> Delay2/1  "colIndex"
  rowCounter/1 -> Delay1/1, Relational Operator/2  "rowIndex"
  enable/1 -> HDL Counter2/2, Logical Operator1/2
  blockLen/1 -> Add/1, Relational Operator1/1
  Constant/1 -> Add/2
  Relational Operator/1 -> Delay/1
  Delay/1 -> colCounter/2, Logical Operator/1
  Logical Operator/1 -> rowCounter/1
  reset/1 -> HDL Counter2/1, Delay15/1
  HDL Counter2/1 -> Relational Operator1/2, Goto/1
  Relational Operator1/1 -> Logical Operator1/1

== system soc_WLAN_fpga/WLAN/WLAN HDL/WLAN_Tx_Rx/WLAN_Rx/WLANHDLReceiver/DataRecovery/Deinterleaver/DeInterleaver_HT/Stage 2 QPSK/Read Logic/Generate Read Address/Read Address of Deinterleaver/Generate Read Address ==
  note: Compute read address
  blockLen : Inport
  enable : Inport  Port=2
  reset : Inport  Port=3
  Add : Sum
  Add1 : Sum  OutDataTypeStr=fixdt(0,nextpow2(maxBlkSize),0)
  Constant : Constant  OutDataTypeStr=fixdt(0,1,0)  SampleTime=-1
  Constant1 : Constant  Value=nColumns-2  OutDataTypeStr=Inherit: Inherit via back propagation  SampleTime=-1
  Constant2 : Constant  Value=nColumns  OutDataTypeStr=fixdt(0,nextpow2(nColumns+1),0)  SampleTime=-1
  Constant4 : Constant  Value=nColumns  OutDataTypeStr=Inherit: Inherit via back propagation  SampleTime=-1
  Delay{,4..6,10..12,14..16} (10 alike) : Delay  DelayLength=1
  Delay{1..3,13} (4 alike) : Delay
  Divide : Product  Inputs=*/  OutDataTypeStr=fixdt(0,nextpow2(maxNRows+1),0)  RndMeth=Zero  SaturateOnIntegerOverflow=on
  From : From
  Goto : Goto
  HDL Counter2 : hdlsllib/Sources/HDL Counter  CountType=Count limited  CountInit=0  CountStep=1  CountMax=maxBlkSize  CountFromType=Initial value  CountFrom=0  CountResetPort=on  CountLoadPort=off  CountEnbPort=on  CountDirPort=off  CountHitOutputPort=off  CountDataType=Unsigned  CountWordLen=nextpow2(maxBlkSize+1)  CountFracLen=0  CountSampTime=1
  Logical Operator : Logic  Operator=OR  IconShape=distinctive  AllPortsSameDT=off  OutDataTypeStr=boolean
  Logical Operator1 : Logic  IconShape=distinctive  AllPortsSameDT=off  OutDataTypeStr=boolean
  Product : Product  OutDataTypeStr=fixdt(0,nextpow2(maxBlkSize),0)
  Relational Operator : RelationalOperator  Operator===  OutDataTypeStr=boolean  InputSameDT=off
  Relational Operator1 : RelationalOperator  OutDataTypeStr=boolean  InputSameDT=off
  Switch : Switch  Criteria=u2 ~= 0  SaturateOnIntegerOverflow=off  InputSameDT=off
  colCounter : hdlsllib/Sources/HDL Counter  CountType=Count limited  CountInit=0  CountStep=1  CountMax=maxNRows -1  CountFromType=Initial value  CountFrom=0  CountResetPort=on  CountLoadPort=off  CountEnbPort=on  CountDirPort=off  CountHitOutputPort=off  CountDataType=Unsigned  CountWordLen=nextpow2(maxNRows)  CountFracLen=0  CountSampTime=1
  rowCounter : hdlsllib/Sources/HDL Counter  CountType=Count limited  CountInit=0  CountStep=1  CountMax=nColumns -1  CountFromType=Initial value  CountFrom=0  CountResetPort=on  CountLoadPort=off  CountEnbPort=on  CountDirPort=off  CountHitOutputPort=off  CountDataType=Unsigned  CountWordLen=nextpow2(nColumns+1)  CountFracLen=0  CountSampTime=1
  blockDataCount : Outport
  currentAddr : Outport  Port=2
  wires:
  Relational Operator1/1 -> Logical Operator1/1
  HDL Counter2/1 -> Goto/1, Relational Operator1/2
  reset/1 -> Delay15/1, HDL Counter2/1
  Logical Operator/1 -> rowCounter/1
  Delay/1 -> Logical Operator/1, colCounter/2
  Relational Operator/1 -> Delay/1
  Constant/1 -> Add/2
  blockLen/1 -> Relational Operator1/1, Add/1
  enable/1 -> Logical Operator1/2, HDL Counter2/2
  rowCounter/1 -> Delay1/1, Relational Operator/2  "rowIndex"
  colCounter/1 -> Delay2/1  "colIndex"
  Add1/1 -> Delay6/1
  Product/1 -> Delay5/1
  Delay2/1 -> Delay4/1
  Delay4/1 -> Add1/2
  Delay5/1 -> Add1/1
  Delay15/1 -> colCounter/1, Logical Operator/2
  Delay16/1 -> Switch/2, rowCounter/2
  Delay13/1 -> Delay14/1
  Delay14/1 -> Delay11/1
  Delay12/1 -> Delay13/1
  Delay6/1 -> currentAddr/1
  Delay11/1 -> blockDataCount/1
  Add/1 -> Delay10/1
  From/1 -> Delay12/1
  Logical Operator1/1 -> Delay16/1
  Divide/1 -> Delay3/1
  Delay10/1 -> Divide/1
  Constant2/1 -> Divide/2
  Switch/1 -> Relational Operator/1
  Constant1/1 -> Switch/1
  Constant4/1 -> Switch/3
  Delay1/1 -> Product/2
  Delay3/1 -> Product/1

== system soc_WLAN_fpga/WLAN/WLAN HDL/WLAN_Tx_Rx/WLAN_Rx/WLANHDLReceiver/DataRecovery/Deinterleaver/DeInterleaver_HT/Stage 2 QPSK/Read Logic/Generate Read Address/Read Address of Interleaver/Generate Read Address ==
  note: Compute read address
  blockLen : Inport
  enable : Inport  Port=2
  reset : Inport  Port=3
  Add : Sum
  Add1 : Sum  Inputs=+-  OutDataTypeStr=Inherit: Inherit via back propagation
  Add2 : Sum  OutDataTypeStr=fixdt(0,nextpow2(maxBlkSize),0)
  Constant : Constant  OutDataTypeStr=fixdt(0,1,0)  SampleTime=-1
  Constant1 : Constant  Value=2  OutDataTypeStr=fixdt(0,2,0)  SampleTime=-1
  Constant2 : Constant  Value=nColumns  OutDataTypeStr=fixdt(0,nextpow2(nColumns+1),0)  SampleTime=-1
  Constant3 : Constant  Value=nColumns  OutDataTypeStr=fixdt(0,nextpow2(nColumns+1),0)  SampleTime=-1
  Constant4 : Constant  Value=maxNRows  OutDataTypeStr=Inherit: Inherit via back propagation  SampleTime=-1
  Delay{,1..16} (17 alike) : Delay  DelayLength=1
  Divide : Product  Inputs=*/  OutDataTypeStr=fixdt(0,nextpow2(maxNRows+1),0)  RndMeth=Zero  SaturateOnIntegerOverflow=on
  From : From
  Goto : Goto
  HDL Counter2 : hdlsllib/Sources/HDL Counter  CountType=Count limited  CountInit=0  CountStep=1  CountMax=maxBlkSize  CountFromType=Initial value  CountFrom=0  CountResetPort=on  CountLoadPort=off  CountEnbPort=on  CountDirPort=off  CountHitOutputPort=off  CountDataType=Unsigned  CountWordLen=nextpow2(maxBlkSize+1)  CountFracLen=0  CountSampTime=1
  Logical Operator : Logic  Operator=OR  IconShape=distinctive  AllPortsSameDT=off  OutDataTypeStr=boolean
  Logical Operator1 : Logic  IconShape=distinctive  AllPortsSameDT=off  OutDataTypeStr=boolean
  Product : Product  OutDataTypeStr=fixdt(0,nextpow2(maxBlkSize),0)
  Relational Operator : RelationalOperator  Operator===  OutDataTypeStr=boolean  InputSameDT=off
  Relational Operator1 : RelationalOperator  OutDataTypeStr=boolean  InputSameDT=off
  Switch : Switch  Criteria=u2 ~= 0  SaturateOnIntegerOverflow=off  InputSameDT=off
  colCounter : hdlsllib/Sources/HDL Counter  CountType=Count limited  CountInit=0  CountStep=1  CountMax=nColumns -1  CountFromType=Initial value  CountFrom=0  CountResetPort=on  CountLoadPort=off  CountEnbPort=on  CountDirPort=off  CountHitOutputPort=off  CountDataType=Unsigned  CountWordLen=nextpow2(nColumns)  CountFracLen=0  CountSampTime=1
  rowCounter : hdlsllib/Sources/HDL Counter  CountType=Count limited  CountInit=0  CountStep=1  CountMax=maxNRows -1  CountFromType=Initial value  CountFrom=0  CountResetPort=on  CountLoadPort=off  CountEnbPort=on  CountDirPort=off  CountHitOutputPort=off  CountDataType=Unsigned  CountWordLen=nextpow2(maxNRows+1)  CountFracLen=0  CountSampTime=1
  blockDataCount : Outport
  currentAddr : Outport  Port=2
  wires:
  Constant3/1 -> Product/2
  Delay9/1 -> Delay13/1
  Delay8/1 -> rowCounter/2, Switch/2
  Delay7/1 -> Logical Operator/2, colCounter/1
  Delay3/1 -> Add1/1
  Delay1/1 -> Product/1
  Add1/1 -> Switch/1
  Constant1/1 -> Add1/2
  Divide/1 -> Delay3/1
  Constant4/1 -> Switch/3
  Switch/1 -> Relational Operator/1
  Constant2/1 -> Divide/2
  Delay10/1 -> Divide/1
  Logical Operator1/1 -> Delay16/1
  From/1 -> Delay12/1
  Add/1 -> Delay10/1
  Delay11/1 -> blockDataCount/1
  Delay6/1 -> currentAddr/1
  Delay12/1 -> Delay9/1
  Delay14/1 -> Delay11/1
  Delay13/1 -> Delay14/1
  Delay16/1 -> Delay8/1
  Delay15/1 -> Delay7/1
  Delay5/1 -> Add2/1
  Delay4/1 -> Add2/2
  Delay2/1 -> Delay4/1
  Product/1 -> Delay5/1
  Add2/1 -> Delay6/1
  colCounter/1 -> Delay2/1  "colIndex"
  rowCounter/1 -> Delay1/1, Relational Operator/2  "rowIndex"
  enable/1 -> HDL Counter2/2, Logical Operator1/2
  blockLen/1 -> Add/1, Relational Operator1/1
  Constant/1 -> Add/2
  Relational Operator/1 -> Delay/1
  Delay/1 -> colCounter/2, Logical Operator/1
  Logical Operator/1 -> rowCounter/1
  reset/1 -> HDL Counter2/1, Delay15/1
  HDL Counter2/1 -> Relational Operator1/2, Goto/1
  Relational Operator1/1 -> Logical Operator1/1

== system soc_WLAN_fpga/WLAN/WLAN HDL/WLAN_Tx_Rx/WLAN_Rx/WLANHDLReceiver/DataRecovery/Deinterleaver/DeInterleaver_NonHT/Stage 2 16QAM /Read Logic/Generate Read Address/Read Address of Deinterleaver/Generate Read Address ==
  note: Compute read address
  blockLen : Inport
  enable : Inport  Port=2
  reset : Inport  Port=3
  Add : Sum
  Add1 : Sum  OutDataTypeStr=fixdt(0,nextpow2(maxBlkSize),0)
  Constant : Constant  OutDataTypeStr=fixdt(0,1,0)  SampleTime=-1
  Constant1 : Constant  Value=nColumns-2  OutDataTypeStr=Inherit: Inherit via back propagation  SampleTime=-1
  Constant2 : Constant  Value=nColumns  OutDataTypeStr=fixdt(0,nextpow2(nColumns+1),0)  SampleTime=-1
  Constant4 : Constant  Value=nColumns  OutDataTypeStr=Inherit: Inherit via back propagation  SampleTime=-1
  Delay{,4..6,10..12,14..16} (10 alike) : Delay  DelayLength=1
  Delay{1..3,13} (4 alike) : Delay
  Divide : Product  Inputs=*/  OutDataTypeStr=fixdt(0,nextpow2(maxNRows+1),0)  RndMeth=Zero  SaturateOnIntegerOverflow=on
  From : From
  Goto : Goto
  HDL Counter2 : hdlsllib/Sources/HDL Counter  CountType=Count limited  CountInit=0  CountStep=1  CountMax=maxBlkSize  CountFromType=Initial value  CountFrom=0  CountResetPort=on  CountLoadPort=off  CountEnbPort=on  CountDirPort=off  CountHitOutputPort=off  CountDataType=Unsigned  CountWordLen=nextpow2(maxBlkSize+1)  CountFracLen=0  CountSampTime=1
  Logical Operator : Logic  Operator=OR  IconShape=distinctive  AllPortsSameDT=off  OutDataTypeStr=boolean
  Logical Operator1 : Logic  IconShape=distinctive  AllPortsSameDT=off  OutDataTypeStr=boolean
  Product : Product  OutDataTypeStr=fixdt(0,nextpow2(maxBlkSize),0)
  Relational Operator : RelationalOperator  Operator===  OutDataTypeStr=boolean  InputSameDT=off
  Relational Operator1 : RelationalOperator  OutDataTypeStr=boolean  InputSameDT=off
  Switch : Switch  Criteria=u2 ~= 0  SaturateOnIntegerOverflow=off  InputSameDT=off
  colCounter : hdlsllib/Sources/HDL Counter  CountType=Count limited  CountInit=0  CountStep=1  CountMax=maxNRows -1  CountFromType=Initial value  CountFrom=0  CountResetPort=on  CountLoadPort=off  CountEnbPort=on  CountDirPort=off  CountHitOutputPort=off  CountDataType=Unsigned  CountWordLen=nextpow2(maxNRows)  CountFracLen=0  CountSampTime=1
  rowCounter : hdlsllib/Sources/HDL Counter  CountType=Count limited  CountInit=0  CountStep=1  CountMax=nColumns -1  CountFromType=Initial value  CountFrom=0  CountResetPort=on  CountLoadPort=off  CountEnbPort=on  CountDirPort=off  CountHitOutputPort=off  CountDataType=Unsigned  CountWordLen=nextpow2(nColumns+1)  CountFracLen=0  CountSampTime=1
  blockDataCount : Outport
  currentAddr : Outport  Port=2
  wires:
  Relational Operator1/1 -> Logical Operator1/1
  HDL Counter2/1 -> Goto/1, Relational Operator1/2
  reset/1 -> Delay15/1, HDL Counter2/1
  Logical Operator/1 -> rowCounter/1
  Delay/1 -> Logical Operator/1, colCounter/2
  Relational Operator/1 -> Delay/1
  Constant/1 -> Add/2
  blockLen/1 -> Relational Operator1/1, Add/1
  enable/1 -> Logical Operator1/2, HDL Counter2/2
  rowCounter/1 -> Delay1/1, Relational Operator/2  "rowIndex"
  colCounter/1 -> Delay2/1  "colIndex"
  Add1/1 -> Delay6/1
  Product/1 -> Delay5/1
  Delay2/1 -> Delay4/1
  Delay4/1 -> Add1/2
  Delay5/1 -> Add1/1
  Delay15/1 -> colCounter/1, Logical Operator/2
  Delay16/1 -> Switch/2, rowCounter/2
  Delay13/1 -> Delay14/1
  Delay14/1 -> Delay11/1
  Delay12/1 -> Delay13/1
  Delay6/1 -> currentAddr/1
  Delay11/1 -> blockDataCount/1
  Add/1 -> Delay10/1
  From/1 -> Delay12/1
  Logical Operator1/1 -> Delay16/1
  Divide/1 -> Delay3/1
  Delay10/1 -> Divide/1
  Constant2/1 -> Divide/2
  Switch/1 -> Relational Operator/1
  Constant1/1 -> Switch/1
  Constant4/1 -> Switch/3
  Delay1/1 -> Product/2
  Delay3/1 -> Product/1

== system soc_WLAN_fpga/WLAN/WLAN HDL/WLAN_Tx_Rx/WLAN_Rx/WLANHDLReceiver/DataRecovery/Deinterleaver/DeInterleaver_NonHT/Stage 2 16QAM /Read Logic/Generate Read Address/Read Address of Interleaver/Generate Read Address ==
  note: Compute read address
  blockLen : Inport
  enable : Inport  Port=2
  reset : Inport  Port=3
  Add : Sum
  Add1 : Sum  Inputs=+-  OutDataTypeStr=Inherit: Inherit via back propagation
  Add2 : Sum  OutDataTypeStr=fixdt(0,nextpow2(maxBlkSize),0)
  Constant : Constant  OutDataTypeStr=fixdt(0,1,0)  SampleTime=-1
  Constant1 : Constant  Value=2  OutDataTypeStr=fixdt(0,2,0)  SampleTime=-1
  Constant2 : Constant  Value=nColumns  OutDataTypeStr=fixdt(0,nextpow2(nColumns+1),0)  SampleTime=-1
  Constant3 : Constant  Value=nColumns  OutDataTypeStr=fixdt(0,nextpow2(nColumns+1),0)  SampleTime=-1
  Constant4 : Constant  Value=maxNRows  OutDataTypeStr=Inherit: Inherit via back propagation  SampleTime=-1
  Delay{,1..16} (17 alike) : Delay  DelayLength=1
  Divide : Product  Inputs=*/  OutDataTypeStr=fixdt(0,nextpow2(maxNRows+1),0)  RndMeth=Zero  SaturateOnIntegerOverflow=on
  From : From
  Goto : Goto
  HDL Counter2 : hdlsllib/Sources/HDL Counter  CountType=Count limited  CountInit=0  CountStep=1  CountMax=maxBlkSize  CountFromType=Initial value  CountFrom=0  CountResetPort=on  CountLoadPort=off  CountEnbPort=on  CountDirPort=off  CountHitOutputPort=off  CountDataType=Unsigned  CountWordLen=nextpow2(maxBlkSize+1)  CountFracLen=0  CountSampTime=1
  Logical Operator : Logic  Operator=OR  IconShape=distinctive  AllPortsSameDT=off  OutDataTypeStr=boolean
  Logical Operator1 : Logic  IconShape=distinctive  AllPortsSameDT=off  OutDataTypeStr=boolean
  Product : Product  OutDataTypeStr=fixdt(0,nextpow2(maxBlkSize),0)
  Relational Operator : RelationalOperator  Operator===  OutDataTypeStr=boolean  InputSameDT=off
  Relational Operator1 : RelationalOperator  OutDataTypeStr=boolean  InputSameDT=off
  Switch : Switch  Criteria=u2 ~= 0  SaturateOnIntegerOverflow=off  InputSameDT=off
  colCounter : hdlsllib/Sources/HDL Counter  CountType=Count limited  CountInit=0  CountStep=1  CountMax=nColumns -1  CountFromType=Initial value  CountFrom=0  CountResetPort=on  CountLoadPort=off  CountEnbPort=on  CountDirPort=off  CountHitOutputPort=off  CountDataType=Unsigned  CountWordLen=nextpow2(nColumns)  CountFracLen=0  CountSampTime=1
  rowCounter : hdlsllib/Sources/HDL Counter  CountType=Count limited  CountInit=0  CountStep=1  CountMax=maxNRows -1  CountFromType=Initial value  CountFrom=0  CountResetPort=on  CountLoadPort=off  CountEnbPort=on  CountDirPort=off  CountHitOutputPort=off  CountDataType=Unsigned  CountWordLen=nextpow2(maxNRows+1)  CountFracLen=0  CountSampTime=1
  blockDataCount : Outport
  currentAddr : Outport  Port=2
  wires:
  Constant3/1 -> Product/2
  Delay9/1 -> Delay13/1
  Delay8/1 -> rowCounter/2, Switch/2
  Delay7/1 -> Logical Operator/2, colCounter/1
  Delay3/1 -> Add1/1
  Delay1/1 -> Product/1
  Add1/1 -> Switch/1
  Constant1/1 -> Add1/2
  Divide/1 -> Delay3/1
  Constant4/1 -> Switch/3
  Switch/1 -> Relational Operator/1
  Constant2/1 -> Divide/2
  Delay10/1 -> Divide/1
  Logical Operator1/1 -> Delay16/1
  From/1 -> Delay12/1
  Add/1 -> Delay10/1
  Delay11/1 -> blockDataCount/1
  Delay6/1 -> currentAddr/1
  Delay12/1 -> Delay9/1
  Delay14/1 -> Delay11/1
  Delay13/1 -> Delay14/1
  Delay16/1 -> Delay8/1
  Delay15/1 -> Delay7/1
  Delay5/1 -> Add2/1
  Delay4/1 -> Add2/2
  Delay2/1 -> Delay4/1
  Product/1 -> Delay5/1
  Add2/1 -> Delay6/1
  colCounter/1 -> Delay2/1  "colIndex"
  rowCounter/1 -> Delay1/1, Relational Operator/2  "rowIndex"
  enable/1 -> HDL Counter2/2, Logical Operator1/2
  blockLen/1 -> Add/1, Relational Operator1/1
  Constant/1 -> Add/2
  Relational Operator/1 -> Delay/1
  Delay/1 -> colCounter/2, Logical Operator/1
  Logical Operator/1 -> rowCounter/1
  reset/1 -> HDL Counter2/1, Delay15/1
  HDL Counter2/1 -> Relational Operator1/2, Goto/1
  Relational Operator1/1 -> Logical Operator1/1
